simulink model "transmission"  (Simulink 7.3)
settings: Solver=ode45  StartTime=0.0  StopTime=0.05  RelTol=1e-3
libraries: powerlib x10, powerlib_extras x1
settings Model: Creator=ss  LastModifiedBy=Sree
settings OptimizationCC: InitFltsAndDblsToZero=on
settings DebuggingCC: SaveWithParameterizedLinksMsg=none  SignalResolutionControl=TryResolveAllWithWarning  MultiTaskDSMMsg=warning  MultiTaskCondExecSysMsg=none
settings RTWCC: IncludeERTFirstTime=on
settings GRTTargetCC: TargetFcnLib=ansi_tfl_tmw.mat

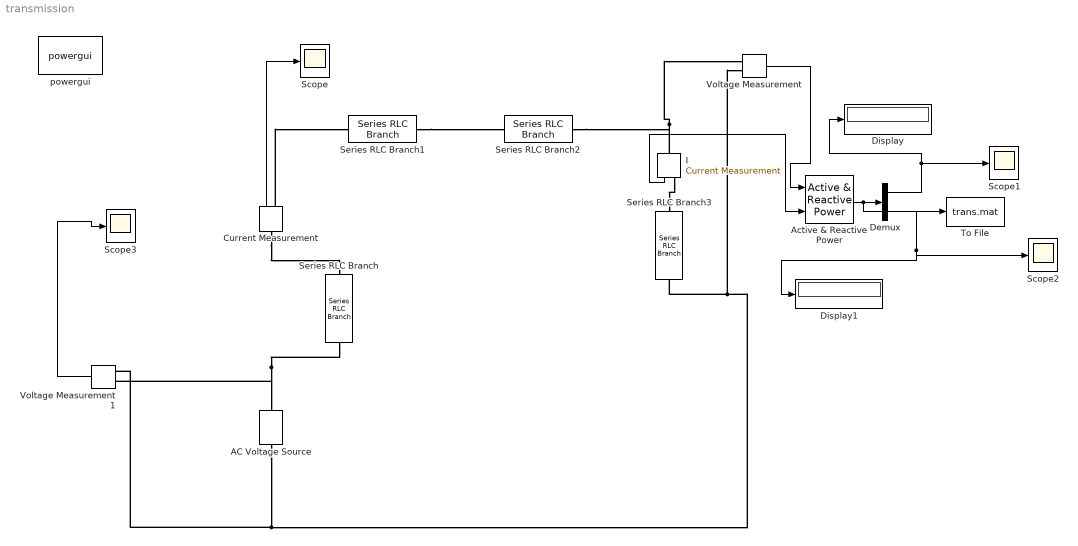
== system transmission ==
  AC Voltage Source : powerlib/Electrical Sources/AC Voltage Source  DialogController=POWERSYS.PowerSysDialog  SystemSampleTime=-1  Amplitude=11000  Phase=0  Frequency=60  SampleTime=0  Measurements=None
  Active & Reactive Power : powerlib_extras/Measurements/Active & Reactive Power  DialogController=POWERSYS.PowerSysDialog  SystemSampleTime=-1  f1=50
  Current Measurement : powerlib/Measurements/Current Measurement  DialogController=POWERSYS.PowerSysDialog  SystemSampleTime=-1  PhasorSimulation=off  OutputType=Complex  PSBequivalent=0
  Demux : Demux  Outputs=2
  Display : Display
  Display1 : Display
  I : powerlib/Measurements/Current Measurement  DialogController=POWERSYS.PowerSysDialog  SystemSampleTime=-1  PhasorSimulation=off  OutputType=Complex  PSBequivalent=0
  Scope{,1..3} (4 alike) : Scope
      Scope settings: TimeRange=0.06  YMin=0  YMax=15  SampleTime=1
      Scope1 settings: TimeRange=0.06  YMin=0  YMax=15  SampleTime=1
      Scope2 settings: TimeRange=0.06  YMin=0  YMax=15  SaveName=ScopeData2  SampleTime=1
      Scope3 settings: TimeRange=0.06  YMin=0  YMax=15  SaveName=ScopeData3  SampleTime=1
  Series RLC Branch : powerlib/Elements/Series RLC Branch  DialogController=POWERSYS.PowerSysDialog  PhysicalDomain=powersysdomain  SubClassName=unknown  LeftPortType=p1  RightPortType=p1  LConnTagsString=__new0  RConnTagsString=__new0  BranchType=RL  Resistance=0.1  Inductance=0.001  SetiL0=off  InitialCurrent=0  Capacitance=1e-6  Setx0=off  InitialVoltage=0  Measurements=Branch voltage
  Series RLC Branch1 : powerlib/Elements/Series RLC Branch  DialogController=POWERSYS.PowerSysDialog  PhysicalDomain=powersysdomain  SubClassName=unknown  LeftPortType=p1  RightPortType=p1  LConnTagsString=__new0  RConnTagsString=__new0  BranchType=RL  Resistance=5  Inductance=0.023  SetiL0=off  InitialCurrent=0  Capacitance=1e-6  Setx0=off  InitialVoltage=0  Measurements=Branch voltage
  Series RLC Branch2 : powerlib/Elements/Series RLC Branch  DialogController=POWERSYS.PowerSysDialog  PhysicalDomain=powersysdomain  SubClassName=unknown  LeftPortType=p1  RightPortType=p1  LConnTagsString=__new0  RConnTagsString=__new0  BranchType=RL  Resistance=5  Inductance=0.023  SetiL0=off  InitialCurrent=0  Capacitance=1e-6  Setx0=off  InitialVoltage=0  Measurements=Branch voltage
  Series RLC Branch3 : powerlib/Elements/Series RLC Branch  DialogController=POWERSYS.PowerSysDialog  PhysicalDomain=powersysdomain  SubClassName=unknown  LeftPortType=p1  RightPortType=p1  LConnTagsString=__new0  RConnTagsString=__new0  BranchType=RL  Resistance=1  Inductance=0.02  SetiL0=off  InitialCurrent=0  Capacitance=1e-6  Setx0=off  InitialVoltage=0  Measurements=Branch voltage
  To File : ToFile  Filename=trans.mat
  Voltage Measurement : powerlib/Measurements/Voltage Measurement  DialogController=POWERSYS.PowerSysDialog  SystemSampleTime=-1  PhasorSimulation=off  OutputType=Complex  PSBequivalent=0
  Voltage Measurement1 : powerlib/Measurements/Voltage Measurement  DialogController=POWERSYS.PowerSysDialog  SystemSampleTime=-1  PhasorSimulation=off  OutputType=Complex  PSBequivalent=0
  powergui : powerlib/powergui  Priority=1  SystemSampleTime=-1  SimulationMode=Continuous  SampleTime=50e-6  frequency=60  SPID=off  DisableSnubberDevices=off  DisableRonSwitches=off  DisableVfSwitches=off  SwTol=0  Interpol=off  frequencyindice=60  echomessages=off  HookPort=off  DisplayEquations=off  FunctionMessages=off  EnableUseOfTLC=off  x0status=blocks  RestoreLinks=warning  Frange=[0:2:500]  Ylog=off  Xlog=on  ShowGrid=off  save=off  variable=ZData  ZoomFFT=off  StartTime=0.0  cycles=1  DisplayStyle=1  fundamental=60  FreqAxis=off  MaxFrequency=1000  frequencyindicesteady=1  RmsSteady=1  display=off  Ts=0  methode=off
  wires:
  Current Measurement/1 -> Scope/1
  Voltage Measurement/1 -> Active & Reactive Power/1
  Active & Reactive Power/1 -> Demux/1, To File/1
  Demux/1 -> Display/1, Scope1/1
  Demux/2 -> Display1/1, Scope2/1
  I/1 -> Active & Reactive Power/2
  Voltage Measurement1/1 -> Scope3/1
  connections:
  Series RLC Branch/RConn1 -- AC Voltage Source/RConn1 -- Voltage Measurement1/LConn1
  Current Measurement/LConn1 -- Series RLC Branch/LConn1
  Current Measurement/RConn1 -- Series RLC Branch1/LConn1
  I/LConn1 -- Voltage Measurement/LConn1 -- Series RLC Branch2/RConn1
  AC Voltage Source/LConn1 -- Series RLC Branch3/RConn1 -- Voltage Measurement/LConn2 -- Voltage Measurement1/LConn2
  I/RConn1 -- Series RLC Branch3/LConn1
  Series RLC Branch1/RConn1 -- Series RLC Branch2/LConn1
